simulink model "adc_sim"  (R2016b)
settings: Solver=VariableStepAuto  StartTime=0.0  StopTime=10.0  RelTol=1e-3
libraries: xps_library x1
settings Model: Creator=qwerty40  LastModifiedBy=qwerty40

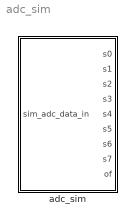
== system adc_sim ==
  adc_sim : Subsystem  mask(adc_sim){nStreams=8, bit_width=8}
      mask prompts: nStreams "Number of Output Streams"; bit_width "Sample Bit Width"
      mask help:
      | This block simulates the behavior of a demuxed ADC, which takes
      | as input a waveform and returns digital samples in parallel at
      | a slower rate.
      |
      | This block is used to simulate the behavior
      mask init:
      | adc_sim_init(gcb, ...
      |     'nStreams', nStreams, ...
      |     'bit_width', bit_width);

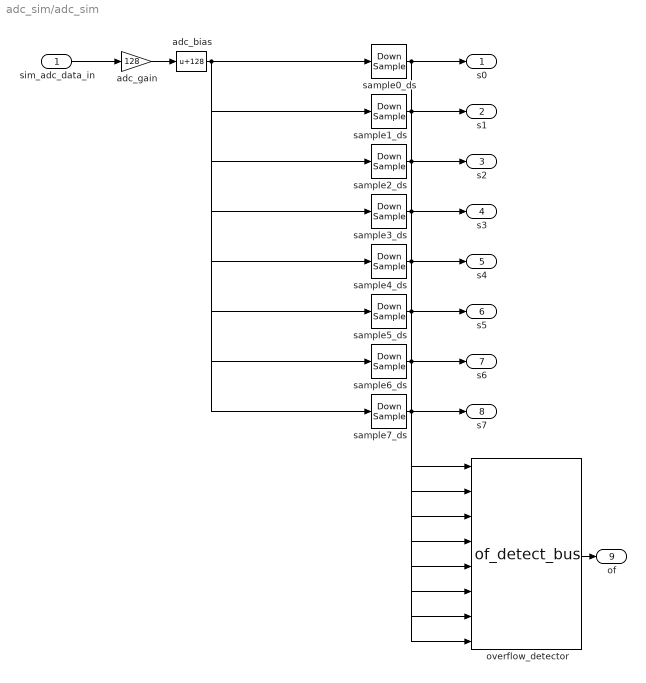
== system adc_sim/adc_sim ==
  sim_adc_data_in : Inport
  adc_bias : Bias  Bias=128  SaturateOnIntegerOverflow=on
  adc_gain : Gain  Gain=128
  overflow_detector : xps_library/ADCs/of_detect_bus  nStreams=8  bit_width=8
  sample0_ds : DownSample  N=8  phase=1  smode=Force single rate
  sample1_ds : DownSample  N=8  phase=2  smode=Force single rate
  sample2_ds : DownSample  N=8  phase=3  smode=Force single rate
  sample3_ds : DownSample  N=8  phase=4  smode=Force single rate
  sample4_ds : DownSample  N=8  phase=5  smode=Force single rate
  sample5_ds : DownSample  N=8  phase=6  smode=Force single rate
  sample6_ds : DownSample  N=8  phase=7  smode=Force single rate
  sample7_ds : DownSample  N=8  smode=Force single rate
  s0 : Outport
  s1 : Outport  Port=2
  s2 : Outport  Port=3
  s3 : Outport  Port=4
  s4 : Outport  Port=5
  s5 : Outport  Port=6
  s6 : Outport  Port=7
  s7 : Outport  Port=8
  of : Outport  Port=9
  wires:
  sample7_ds/1 -> s7/1, overflow_detector/8
  sample6_ds/1 -> s6/1, overflow_detector/7
  sample5_ds/1 -> s5/1, overflow_detector/6
  sample4_ds/1 -> s4/1, overflow_detector/5
  sample3_ds/1 -> s3/1, overflow_detector/4
  sample2_ds/1 -> s2/1, overflow_detector/3
  sample1_ds/1 -> s1/1, overflow_detector/2
  sample0_ds/1 -> s0/1, overflow_detector/1
  adc_bias/1 -> sample7_ds/1, sample6_ds/1, sample5_ds/1, sample4_ds/1, sample3_ds/1, sample2_ds/1, sample1_ds/1, sample0_ds/1
  overflow_detector/1 -> of/1
  adc_gain/1 -> adc_bias/1
  sim_adc_data_in/1 -> adc_gain/1
